simulink model "Expt1"  (R2023b)
settings: Solver=VariableStepAuto  StartTime=0.0  StopTime=0.1  RelTol=1e-3  AbsTol=1e-3
libraries: spsRMSLib x8, eePowerMeasurement x6, spsVoltageMeasurementLib x6, spsSeriesRLCBranchLib x4, spsACVoltageSourceLib x2, spsCurrentMeasurementLib x2, spspowerguiLib x1
settings Model: Creator=anand  LastModifiedBy=anand
settings SolverCC: AutoScaleAbsTol=off  AlgebraicLoopSolver=TrustRegion  MaxZcPerStep=1
settings DebuggingCC: UnconnectedInputMsg=warning  UnconnectedOutputMsg=warning  UnconnectedLineMsg=warning  SymbolicDimsDataTypeCodeGenerationDiagnostic=none
settings ModelReferenceCC: EnableRefExpFcnMdlSchedulingChecks=on
settings SFSimCC: CustomCodeUndefinedFunction=UseInterfaceOnly
settings RTWCC: DLArmComputeVersion=19.05
settings SimscapeCC: SimscapeLogType=all  SimscapeLogSimulationStatistics=on  SimscapeLogDataHistory=10000

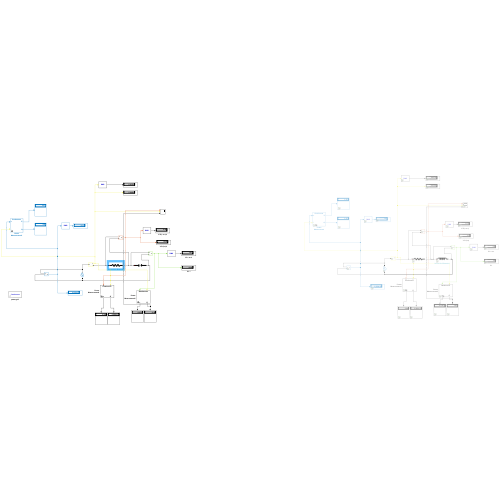
[thumbnail: Simulink's stored preview of the top-level diagram]
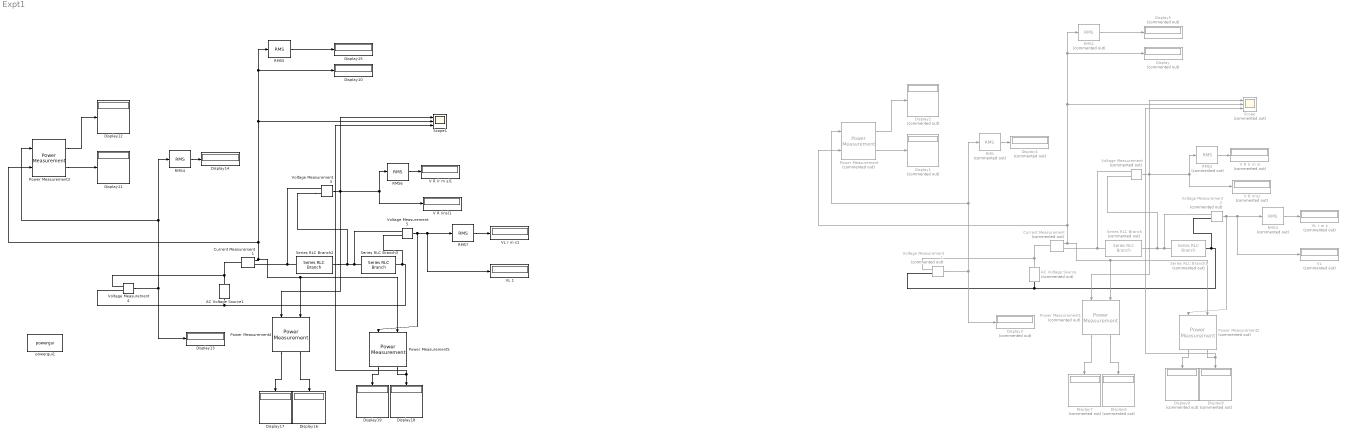
== system Expt1 ==
  AC Voltage Source : spsACVoltageSourceLib/AC Voltage Source  Commented=on  Amplitude=220  Phase=0  Frequency=50  SampleTime=0  Measurements=None  BusType=swing  Pref=10e3  Qref=0  Qmin=-inf  Qmax=+inf
  AC Voltage Source1 : spsACVoltageSourceLib/AC Voltage Source  Amplitude=220  Phase=0  Frequency=50  SampleTime=0  Measurements=None  BusType=swing  Pref=10e3  Qref=0  Qmin=-inf  Qmax=+inf
  Current Measurement : spsCurrentMeasurementLib/Current Measurement  Commented=on  PhasorSimulation=off  OutputType=Complex  PSBequivalent=0
  Current Measurement1 : spsCurrentMeasurementLib/Current Measurement  PhasorSimulation=off  OutputType=Complex  PSBequivalent=0
  Display{,1..9} (10 alike) : Display  Commented=on
  Display{10..19} (10 alike) : Display
  Power Measurement : eePowerMeasurement/Power Measurement  Commented=on  LabelModeActiveChoice=Continuous  F=50  K=[1]  Ts=0
  Power Measurement1 : eePowerMeasurement/Power Measurement  Commented=on  LabelModeActiveChoice=Continuous  F=50  K=[1]  Ts=0
  Power Measurement2 : eePowerMeasurement/Power Measurement  Commented=on  LabelModeActiveChoice=Continuous  F=50  K=[1]  Ts=0
  Power Measurement3 : eePowerMeasurement/Power Measurement  LabelModeActiveChoice=Continuous  F=50  K=[1]  Ts=0
  Power Measurement4 : eePowerMeasurement/Power Measurement  LabelModeActiveChoice=Continuous  F=50  K=[1]  Ts=0
  Power Measurement5 : eePowerMeasurement/Power Measurement  LabelModeActiveChoice=Continuous  F=50  K=[1]  Ts=0
  RMS{,1..3} (4 alike) : spsRMSLib/RMS  Commented=on  TrueRMS=on  Freq=60  RMSInit=120  Ts=0
  RMS{4..7} (4 alike) : spsRMSLib/RMS  TrueRMS=on  Freq=60  RMSInit=120  Ts=0
  Scope : Scope  Commented=on  NumInputPorts=3
  Scope1 : Scope  NumInputPorts=3
  Series RLC Branch : spsSeriesRLCBranchLib/Series RLC Branch  Commented=on  LConnTagsString=__new0  RConnTagsString=__new0  BranchType=R  Resistance=3140  Inductance=1e-1  SetiL0=off  InitialCurrent=0  Capacitance=1e-2  Setx0=off  InitialVoltage=0  Measurements=None
  Series RLC Branch1 : spsSeriesRLCBranchLib/Series RLC Branch  Commented=on  LConnTagsString=__new0  RConnTagsString=__new0  BranchType=L  Resistance=1  Inductance=10  SetiL0=off  InitialCurrent=0  Capacitance=1e-6  Setx0=off  InitialVoltage=0  Measurements=None
  Series RLC Branch2 : spsSeriesRLCBranchLib/Series RLC Branch  LConnTagsString=__new0  RConnTagsString=__new0  BranchType=R  Resistance=2000  Inductance=1e-1  SetiL0=off  InitialCurrent=0  Capacitance=1e-2  Setx0=off  InitialVoltage=0  Measurements=None
  Series RLC Branch3 : spsSeriesRLCBranchLib/Series RLC Branch  LConnTagsString=__new0  RConnTagsString=__new0  BranchType=C  Resistance=1  Inductance=10  SetiL0=off  InitialCurrent=0  Capacitance=1e-6  Setx0=off  InitialVoltage=0  Measurements=None
  V R (ins) : Display  Commented=on
  V R (ins)1 : Display
  V R (r m s) : Display  Commented=on
  V R (r m s)1 : Display
  "VL " : Display  Commented=on
  VL 1 : Display
  VL r m s : Display  Commented=on
  VL r m s1 : Display
  Voltage Measurement : spsVoltageMeasurementLib/Voltage Measurement  Commented=on  PhasorSimulation=off  OutputType=Complex  PSBequivalent=0
  Voltage Measurement1 : spsVoltageMeasurementLib/Voltage Measurement  Commented=on  PhasorSimulation=off  OutputType=Complex  PSBequivalent=0
  Voltage Measurement2 : spsVoltageMeasurementLib/Voltage Measurement  Commented=on  PhasorSimulation=off  OutputType=Complex  PSBequivalent=0
  Voltage Measurement3 : spsVoltageMeasurementLib/Voltage Measurement  PhasorSimulation=off  OutputType=Complex  PSBequivalent=0
  Voltage Measurement4 : spsVoltageMeasurementLib/Voltage Measurement  PhasorSimulation=off  OutputType=Complex  PSBequivalent=0
  Voltage Measurement5 : spsVoltageMeasurementLib/Voltage Measurement  PhasorSimulation=off  OutputType=Complex  PSBequivalent=0
  powergui1 : spspowerguiLib/powergui  Priority=1  SimulationMode=Continuous  SampleTime=50e-6  frequency=60  Iterations=50  frequencyindice=50  Pbase=100e6  ErrMax=1e-4  UnitsV=kV  UnitsW=MW  buscounter=0  FunctionMessages=off  echomessages=off  EnableUseOfTLC=off  CurrentSourceSwitches=off  DisableSnubberDevices=off  DisableRonSwitches=off  DisableVfSwitches=off  DisplayEquations=off  AutomaticDiscreteSolvers=off  SolverType=Tustin/Backward Euler (TBE)  Interpol=off  ExternalGateDelay=off  methode=off  Ts=100  x0status=blocks  SPID=on  SwTol=0  HookPort=off  NonlinearTolerance=1e-4  nMaxIteration=100  ContinueOnMaxIteration=off  RestoreLinks=warning  ResistiveCurrentMeasurement=off  Frange=[0:2:500]  Ylog=off  Xlog=on  ShowGrid=off  save=off  variable=ZData  structure=0  ZoomFFT=off  StartTime=0.0  cycles=1  DisplayStyle=1  fundamental=60  FreqAxis=off  MaxFrequency=1000  frequencyindicesteady=1  RmsSteady=1  display=off
  wires:
  Voltage Measurement/1 -> Scope/1, Power Measurement1/1, RMS2/1, V R (ins)/1
  Voltage Measurement1/1 -> RMS/1, Power Measurement/1, Display3/1
  RMS/1 -> Display4/1
  RMS1/1 -> Display5/1
  RMS2/1 -> V R (r m s)/1
  RMS3/1 -> VL r m s/1
  Power Measurement/1 -> Display2/1
  Power Measurement/2 -> Display1/1
  Power Measurement1/1 -> Display7/1
  Power Measurement1/2 -> Display6/1
  Power Measurement2/1 -> Display9/1
  Power Measurement2/2 -> Display8/1, Scope/3
  Current Measurement/1 -> Power Measurement2/2, Power Measurement1/2, Scope/2, RMS1/1, Display/1, Power Measurement/2
  Voltage Measurement2/1 -> Power Measurement2/1, "VL "/1, RMS3/1
  Power Measurement5/1 -> Display19/1
  RMS5/1 -> Display15/1
  Power Measurement5/2 -> Display18/1, Scope1/3
  Power Measurement4/2 -> Display16/1
  Power Measurement4/1 -> Display17/1
  Power Measurement3/2 -> Display11/1
  Power Measurement3/1 -> Display12/1
  RMS6/1 -> V R (r m s)1/1
  Voltage Measurement5/1 -> Power Measurement5/1, VL 1/1, RMS7/1
  RMS4/1 -> Display14/1
  RMS7/1 -> VL r m s1/1
  Current Measurement1/1 -> Power Measurement5/2, Power Measurement4/2, Scope1/2, RMS5/1, Display10/1, Power Measurement3/2
  Voltage Measurement4/1 -> RMS4/1, Power Measurement3/1, Display13/1
  Voltage Measurement3/1 -> Scope1/1, Power Measurement4/1, RMS6/1, V R (ins)1/1
  connections:
  Series RLC Branch/LConn1 -- Voltage Measurement/LConn1 -- Current Measurement/RConn1
  Current Measurement/LConn1 -- Voltage Measurement1/LConn1 -- AC Voltage Source/RConn1
  AC Voltage Source/LConn1 -- Voltage Measurement1/LConn2 -- Voltage Measurement2/LConn2 -- Series RLC Branch1/RConn1
  Series RLC Branch1/LConn1 -- Voltage Measurement2/LConn1 -- Series RLC Branch/RConn1 -- Voltage Measurement/LConn2
  AC Voltage Source1/LConn1 -- Voltage Measurement4/LConn2 -- Voltage Measurement5/LConn2 -- Series RLC Branch3/RConn1
  Voltage Measurement3/LConn2 -- Series RLC Branch3/LConn1 -- Voltage Measurement5/LConn1 -- Series RLC Branch2/RConn1
  Current Measurement1/RConn1 -- Series RLC Branch2/LConn1 -- Voltage Measurement3/LConn1
  AC Voltage Source1/RConn1 -- Current Measurement1/LConn1 -- Voltage Measurement4/LConn1
